simulink model "xEMU_SimulationModel3_rule1"  (R2017b)
settings: Solver=ode4  StartTime=0.0  StopTime=8192  FixedStep=0.01  RelTol=1e-3
undefined symbols (not defined in the file): a1, a2, a3, a4, ACO, BAT, Battery, DCT, DRT, EMS, ENV, Fahrzyklus_VS_modell, height_BAT, leistung, lib_bat, Maximum, Maximum_position, Num_cells, P_FC_max_long, P_FC_min_long, P_FC_step_max, Pbat_charge_max, Pbat_discharge_max, Pfc_max, Pfc_min, SOC_tar, time_peaks, TRM, velocity_peaks
libraries: simulink x5
(part 6 of 15)

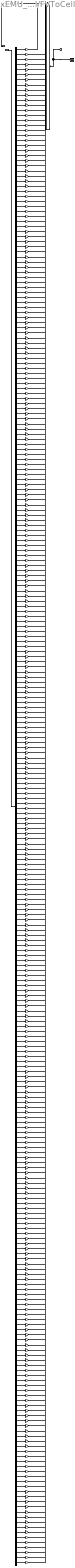
== system xEMU_SimulationModel3_rule1/Battery (BAT)_mittel/Battery/Thermal/FVToCell ==
  T_FV : Inport
  AddCell1 : Sum  Inputs=<binary blob, 300 chars, not shown>
  Demux : Demux  Outputs=300
  Scope : Scope
  T_FV_{1..300} (300 alike) : Gain  Gain=0.0033333  SaturateOnIntegerOverflow=on  OutDataTypeStr=Inherit: Same as input  ParamDataTypeStr=Inherit: Same as input
  Out1 : Outport
  tag scope: T_CellElement1=scoped
  wires:
  T_FV/1 -> Demux/1
  Demux/1 -> T_FV_1/1
  Demux/2 -> T_FV_2/1
  Demux/3 -> T_FV_3/1
  Demux/4 -> T_FV_4/1
  Demux/5 -> T_FV_5/1
  Demux/6 -> T_FV_6/1
  Demux/7 -> T_FV_7/1
  Demux/8 -> T_FV_8/1
  Demux/9 -> T_FV_9/1
  Demux/10 -> T_FV_10/1
  Demux/11 -> T_FV_11/1
  Demux/12 -> T_FV_12/1
  Demux/13 -> T_FV_13/1
  Demux/14 -> T_FV_14/1
  Demux/15 -> T_FV_15/1
  Demux/16 -> T_FV_16/1
  Demux/17 -> T_FV_17/1
  Demux/18 -> T_FV_18/1
  Demux/19 -> T_FV_19/1
  Demux/20 -> T_FV_20/1
  Demux/21 -> T_FV_21/1
  Demux/22 -> T_FV_22/1
  Demux/23 -> T_FV_23/1
  Demux/24 -> T_FV_24/1
  Demux/25 -> T_FV_25/1
  Demux/26 -> T_FV_26/1
  Demux/27 -> T_FV_27/1
  Demux/28 -> T_FV_28/1
  Demux/29 -> T_FV_29/1
  Demux/30 -> T_FV_30/1
  Demux/31 -> T_FV_31/1
  Demux/32 -> T_FV_32/1
  Demux/33 -> T_FV_33/1
  Demux/34 -> T_FV_34/1
  Demux/35 -> T_FV_35/1
  Demux/36 -> T_FV_36/1
  Demux/37 -> T_FV_37/1
  Demux/38 -> T_FV_38/1
  Demux/39 -> T_FV_39/1
  Demux/40 -> T_FV_40/1
  Demux/41 -> T_FV_41/1
  Demux/42 -> T_FV_42/1
  Demux/43 -> T_FV_43/1
  Demux/44 -> T_FV_44/1
  Demux/45 -> T_FV_45/1
  Demux/46 -> T_FV_46/1
  Demux/47 -> T_FV_47/1
  Demux/48 -> T_FV_48/1
  Demux/49 -> T_FV_49/1
  Demux/50 -> T_FV_50/1
  Demux/51 -> T_FV_51/1
  Demux/52 -> T_FV_52/1
  Demux/53 -> T_FV_53/1
  Demux/54 -> T_FV_54/1
  Demux/55 -> T_FV_55/1
  Demux/56 -> T_FV_56/1
  Demux/57 -> T_FV_57/1
  Demux/58 -> T_FV_58/1
  Demux/59 -> T_FV_59/1
  Demux/60 -> T_FV_60/1
  Demux/61 -> T_FV_61/1
  Demux/62 -> T_FV_62/1
  Demux/63 -> T_FV_63/1
  Demux/64 -> T_FV_64/1
  Demux/65 -> T_FV_65/1
  Demux/66 -> T_FV_66/1
  Demux/67 -> T_FV_67/1
  Demux/68 -> T_FV_68/1
  Demux/69 -> T_FV_69/1
  Demux/70 -> T_FV_70/1
  Demux/71 -> T_FV_71/1
  Demux/72 -> T_FV_72/1
  Demux/73 -> T_FV_73/1
  Demux/74 -> T_FV_74/1
  Demux/75 -> T_FV_75/1
  Demux/76 -> T_FV_76/1
  Demux/77 -> T_FV_77/1
  Demux/78 -> T_FV_78/1
  Demux/79 -> T_FV_79/1
  Demux/80 -> T_FV_80/1
  Demux/81 -> T_FV_81/1
  Demux/82 -> T_FV_82/1
  Demux/83 -> T_FV_83/1
  Demux/84 -> T_FV_84/1
  Demux/85 -> T_FV_85/1
  Demux/86 -> T_FV_86/1
  Demux/87 -> T_FV_87/1
  Demux/88 -> T_FV_88/1
  Demux/89 -> T_FV_89/1
  Demux/90 -> T_FV_90/1
  Demux/91 -> T_FV_91/1
  Demux/92 -> T_FV_92/1
  Demux/93 -> T_FV_93/1
  Demux/94 -> T_FV_94/1
  Demux/95 -> T_FV_95/1
  Demux/96 -> T_FV_96/1
  Demux/97 -> T_FV_97/1
  Demux/98 -> T_FV_98/1
  Demux/99 -> T_FV_99/1
  Demux/100 -> T_FV_100/1
  Demux/101 -> T_FV_101/1
  Demux/102 -> T_FV_102/1
  Demux/103 -> T_FV_103/1
  Demux/104 -> T_FV_104/1
  Demux/105 -> T_FV_105/1
  Demux/106 -> T_FV_106/1
  Demux/107 -> T_FV_107/1
  Demux/108 -> T_FV_108/1
  Demux/109 -> T_FV_109/1
  Demux/110 -> T_FV_110/1
  Demux/111 -> T_FV_111/1
  Demux/112 -> T_FV_112/1
  Demux/113 -> T_FV_113/1
  Demux/114 -> T_FV_114/1
  Demux/115 -> T_FV_115/1
  Demux/116 -> T_FV_116/1
  Demux/117 -> T_FV_117/1
  Demux/118 -> T_FV_118/1
  Demux/119 -> T_FV_119/1
  Demux/120 -> T_FV_120/1
  Demux/121 -> T_FV_121/1
  Demux/122 -> T_FV_122/1
  Demux/123 -> T_FV_123/1
  Demux/124 -> T_FV_124/1
  Demux/125 -> T_FV_125/1
  Demux/126 -> T_FV_126/1
  Demux/127 -> T_FV_127/1
  Demux/128 -> T_FV_128/1
  Demux/129 -> T_FV_129/1
  Demux/130 -> T_FV_130/1
  Demux/131 -> T_FV_131/1
  Demux/132 -> T_FV_132/1
  Demux/133 -> T_FV_133/1
  Demux/134 -> T_FV_134/1
  Demux/135 -> T_FV_135/1
  Demux/136 -> T_FV_136/1
  Demux/137 -> T_FV_137/1
  Demux/138 -> T_FV_138/1
  Demux/139 -> T_FV_139/1
  Demux/140 -> T_FV_140/1
  Demux/141 -> T_FV_141/1
  Demux/142 -> T_FV_142/1
  Demux/143 -> T_FV_143/1
  Demux/144 -> T_FV_144/1
  Demux/145 -> T_FV_145/1
  Demux/146 -> T_FV_146/1
  Demux/147 -> T_FV_147/1
  Demux/148 -> T_FV_148/1
  Demux/149 -> T_FV_149/1
  Demux/150 -> T_FV_150/1
  Demux/151 -> T_FV_151/1
  Demux/152 -> T_FV_152/1
  Demux/153 -> T_FV_153/1
  Demux/154 -> T_FV_154/1
  Demux/155 -> T_FV_155/1
  Demux/156 -> T_FV_156/1
  Demux/157 -> T_FV_157/1
  Demux/158 -> T_FV_158/1
  Demux/159 -> T_FV_159/1
  Demux/160 -> T_FV_160/1
  Demux/161 -> T_FV_161/1
  Demux/162 -> T_FV_162/1
  Demux/163 -> T_FV_163/1
  Demux/164 -> T_FV_164/1
  Demux/165 -> T_FV_165/1
  Demux/166 -> T_FV_166/1
  Demux/167 -> T_FV_167/1
  Demux/168 -> T_FV_168/1
  Demux/169 -> T_FV_169/1
  Demux/170 -> T_FV_170/1
  Demux/171 -> T_FV_171/1
  Demux/172 -> T_FV_172/1
  Demux/173 -> T_FV_173/1
  Demux/174 -> T_FV_174/1
  Demux/175 -> T_FV_175/1
  Demux/176 -> T_FV_176/1
  Demux/177 -> T_FV_177/1
  Demux/178 -> T_FV_178/1
  Demux/179 -> T_FV_179/1
  Demux/180 -> T_FV_180/1
  Demux/181 -> T_FV_181/1
  Demux/182 -> T_FV_182/1
  Demux/183 -> T_FV_183/1
  Demux/184 -> T_FV_184/1
  Demux/185 -> T_FV_185/1
  Demux/186 -> T_FV_186/1
  Demux/187 -> T_FV_187/1
  Demux/188 -> T_FV_188/1
  Demux/189 -> T_FV_189/1
  Demux/190 -> T_FV_190/1
  Demux/191 -> T_FV_191/1
  Demux/192 -> T_FV_192/1
  Demux/193 -> T_FV_193/1
  Demux/194 -> T_FV_194/1
  Demux/195 -> T_FV_195/1
  Demux/196 -> T_FV_196/1
  Demux/197 -> T_FV_197/1
  Demux/198 -> T_FV_198/1
  Demux/199 -> T_FV_199/1
  Demux/200 -> T_FV_200/1
  Demux/201 -> T_FV_201/1
  Demux/202 -> T_FV_202/1
  Demux/203 -> T_FV_203/1
  Demux/204 -> T_FV_204/1
  Demux/205 -> T_FV_205/1
  Demux/206 -> T_FV_206/1
  Demux/207 -> T_FV_207/1
  Demux/208 -> T_FV_208/1
  Demux/209 -> T_FV_209/1
  Demux/210 -> T_FV_210/1
  Demux/211 -> T_FV_211/1
  Demux/212 -> T_FV_212/1
  Demux/213 -> T_FV_213/1
  Demux/214 -> T_FV_214/1
  Demux/215 -> T_FV_215/1
  Demux/216 -> T_FV_216/1
  Demux/217 -> T_FV_217/1
  Demux/218 -> T_FV_218/1
  Demux/219 -> T_FV_219/1
  Demux/220 -> T_FV_220/1
  Demux/221 -> T_FV_221/1
  Demux/222 -> T_FV_222/1
  Demux/223 -> T_FV_223/1
  Demux/224 -> T_FV_224/1
  Demux/225 -> T_FV_225/1
  Demux/226 -> T_FV_226/1
  Demux/227 -> T_FV_227/1
  Demux/228 -> T_FV_228/1
  Demux/229 -> T_FV_229/1
  Demux/230 -> T_FV_230/1
  Demux/231 -> T_FV_231/1
  Demux/232 -> T_FV_232/1
  Demux/233 -> T_FV_233/1
  Demux/234 -> T_FV_234/1
  Demux/235 -> T_FV_235/1
  Demux/236 -> T_FV_236/1
  Demux/237 -> T_FV_237/1
  Demux/238 -> T_FV_238/1
  Demux/239 -> T_FV_239/1
  Demux/240 -> T_FV_240/1
  Demux/241 -> T_FV_241/1
  Demux/242 -> T_FV_242/1
  Demux/243 -> T_FV_243/1
  Demux/244 -> T_FV_244/1
  Demux/245 -> T_FV_245/1
  Demux/246 -> T_FV_246/1
  Demux/247 -> T_FV_247/1
  Demux/248 -> T_FV_248/1
  Demux/249 -> T_FV_249/1
  Demux/250 -> T_FV_250/1
  Demux/251 -> T_FV_251/1
  Demux/252 -> T_FV_252/1
  Demux/253 -> T_FV_253/1
  Demux/254 -> T_FV_254/1
  Demux/255 -> T_FV_255/1
  Demux/256 -> T_FV_256/1
  Demux/257 -> T_FV_257/1
  Demux/258 -> T_FV_258/1
  Demux/259 -> T_FV_259/1
  Demux/260 -> T_FV_260/1
  Demux/261 -> T_FV_261/1
  Demux/262 -> T_FV_262/1
  Demux/263 -> T_FV_263/1
  Demux/264 -> T_FV_264/1
  Demux/265 -> T_FV_265/1
  Demux/266 -> T_FV_266/1
  Demux/267 -> T_FV_267/1
  Demux/268 -> T_FV_268/1
  Demux/269 -> T_FV_269/1
  Demux/270 -> T_FV_270/1
  Demux/271 -> T_FV_271/1
  Demux/272 -> T_FV_272/1
  Demux/273 -> T_FV_273/1
  Demux/274 -> T_FV_274/1
  Demux/275 -> T_FV_275/1
  Demux/276 -> T_FV_276/1
  Demux/277 -> T_FV_277/1
  Demux/278 -> T_FV_278/1
  Demux/279 -> T_FV_279/1
  Demux/280 -> T_FV_280/1
  Demux/281 -> T_FV_281/1
  Demux/282 -> T_FV_282/1
  Demux/283 -> T_FV_283/1
  Demux/284 -> T_FV_284/1
  Demux/285 -> T_FV_285/1
  Demux/286 -> T_FV_286/1
  Demux/287 -> T_FV_287/1
  Demux/288 -> T_FV_288/1
  Demux/289 -> T_FV_289/1
  Demux/290 -> T_FV_290/1
  Demux/291 -> T_FV_291/1
  Demux/292 -> T_FV_292/1
  Demux/293 -> T_FV_293/1
  Demux/294 -> T_FV_294/1
  Demux/295 -> T_FV_295/1
  Demux/296 -> T_FV_296/1
  Demux/297 -> T_FV_297/1
  Demux/298 -> T_FV_298/1
  Demux/299 -> T_FV_299/1
  Demux/300 -> T_FV_300/1
  AddCell1/1 -> Scope/1, [T_CellElement1], Out1/1
  T_FV_1/1 -> AddCell1/1
  T_FV_2/1 -> AddCell1/2
  T_FV_3/1 -> AddCell1/3
  T_FV_4/1 -> AddCell1/4
  T_FV_5/1 -> AddCell1/5
  T_FV_6/1 -> AddCell1/6
  T_FV_7/1 -> AddCell1/7
  T_FV_8/1 -> AddCell1/8
  T_FV_9/1 -> AddCell1/9
  T_FV_10/1 -> AddCell1/10
  T_FV_11/1 -> AddCell1/11
  T_FV_12/1 -> AddCell1/12
  T_FV_13/1 -> AddCell1/13
  T_FV_14/1 -> AddCell1/14
  T_FV_15/1 -> AddCell1/15
  T_FV_16/1 -> AddCell1/16
  T_FV_17/1 -> AddCell1/17
  T_FV_18/1 -> AddCell1/18
  T_FV_19/1 -> AddCell1/19
  T_FV_20/1 -> AddCell1/20
  T_FV_21/1 -> AddCell1/21
  T_FV_22/1 -> AddCell1/22
  T_FV_23/1 -> AddCell1/23
  T_FV_24/1 -> AddCell1/24
  T_FV_25/1 -> AddCell1/25
  T_FV_26/1 -> AddCell1/26
  T_FV_27/1 -> AddCell1/27
  T_FV_28/1 -> AddCell1/28
  T_FV_29/1 -> AddCell1/29
  T_FV_30/1 -> AddCell1/30
  T_FV_31/1 -> AddCell1/31
  T_FV_32/1 -> AddCell1/32
  T_FV_33/1 -> AddCell1/33
  T_FV_34/1 -> AddCell1/34
  T_FV_35/1 -> AddCell1/35
  T_FV_36/1 -> AddCell1/36
  T_FV_37/1 -> AddCell1/37
  T_FV_38/1 -> AddCell1/38
  T_FV_39/1 -> AddCell1/39
  T_FV_40/1 -> AddCell1/40
  T_FV_41/1 -> AddCell1/41
  T_FV_42/1 -> AddCell1/42
  T_FV_43/1 -> AddCell1/43
  T_FV_44/1 -> AddCell1/44
  T_FV_45/1 -> AddCell1/45
  T_FV_46/1 -> AddCell1/46
  T_FV_47/1 -> AddCell1/47
  T_FV_48/1 -> AddCell1/48
  T_FV_49/1 -> AddCell1/49
  T_FV_50/1 -> AddCell1/50
  T_FV_51/1 -> AddCell1/51
  T_FV_52/1 -> AddCell1/52
  T_FV_53/1 -> AddCell1/53
  T_FV_54/1 -> AddCell1/54
  T_FV_55/1 -> AddCell1/55
  T_FV_56/1 -> AddCell1/56
  T_FV_57/1 -> AddCell1/57
  T_FV_58/1 -> AddCell1/58
  T_FV_59/1 -> AddCell1/59
  T_FV_60/1 -> AddCell1/60
  T_FV_61/1 -> AddCell1/61
  T_FV_62/1 -> AddCell1/62
  T_FV_63/1 -> AddCell1/63
  T_FV_64/1 -> AddCell1/64
  T_FV_65/1 -> AddCell1/65
  T_FV_66/1 -> AddCell1/66
  T_FV_67/1 -> AddCell1/67
  T_FV_68/1 -> AddCell1/68
  T_FV_69/1 -> AddCell1/69
  T_FV_70/1 -> AddCell1/70
  T_FV_71/1 -> AddCell1/71
  T_FV_72/1 -> AddCell1/72
  T_FV_73/1 -> AddCell1/73
  T_FV_74/1 -> AddCell1/74
  T_FV_75/1 -> AddCell1/75
  T_FV_76/1 -> AddCell1/76
  T_FV_77/1 -> AddCell1/77
  T_FV_78/1 -> AddCell1/78
  T_FV_79/1 -> AddCell1/79
  T_FV_80/1 -> AddCell1/80
  T_FV_81/1 -> AddCell1/81
  T_FV_82/1 -> AddCell1/82
  T_FV_83/1 -> AddCell1/83
  T_FV_84/1 -> AddCell1/84
  T_FV_85/1 -> AddCell1/85
  T_FV_86/1 -> AddCell1/86
  T_FV_87/1 -> AddCell1/87
  T_FV_88/1 -> AddCell1/88
  T_FV_89/1 -> AddCell1/89
  T_FV_90/1 -> AddCell1/90
  T_FV_91/1 -> AddCell1/91
  T_FV_92/1 -> AddCell1/92
  T_FV_93/1 -> AddCell1/93
  T_FV_94/1 -> AddCell1/94
  T_FV_95/1 -> AddCell1/95
  T_FV_96/1 -> AddCell1/96
  T_FV_97/1 -> AddCell1/97
  T_FV_98/1 -> AddCell1/98
  T_FV_99/1 -> AddCell1/99
  T_FV_100/1 -> AddCell1/100
  T_FV_101/1 -> AddCell1/101
  T_FV_102/1 -> AddCell1/102
  T_FV_103/1 -> AddCell1/103
  T_FV_104/1 -> AddCell1/104
  T_FV_105/1 -> AddCell1/105
  T_FV_106/1 -> AddCell1/106
  T_FV_107/1 -> AddCell1/107
  T_FV_108/1 -> AddCell1/108
  T_FV_109/1 -> AddCell1/109
  T_FV_110/1 -> AddCell1/110
  T_FV_111/1 -> AddCell1/111
  T_FV_112/1 -> AddCell1/112
  T_FV_113/1 -> AddCell1/113
  T_FV_114/1 -> AddCell1/114
  T_FV_115/1 -> AddCell1/115
  T_FV_116/1 -> AddCell1/116
  T_FV_117/1 -> AddCell1/117
  T_FV_118/1 -> AddCell1/118
  T_FV_119/1 -> AddCell1/119
  T_FV_120/1 -> AddCell1/120
  T_FV_121/1 -> AddCell1/121
  T_FV_122/1 -> AddCell1/122
  T_FV_123/1 -> AddCell1/123
  T_FV_124/1 -> AddCell1/124
  T_FV_125/1 -> AddCell1/125
  T_FV_126/1 -> AddCell1/126
  T_FV_127/1 -> AddCell1/127
  T_FV_128/1 -> AddCell1/128
  T_FV_129/1 -> AddCell1/129
  T_FV_130/1 -> AddCell1/130
  T_FV_131/1 -> AddCell1/131
  T_FV_132/1 -> AddCell1/132
  T_FV_133/1 -> AddCell1/133
  T_FV_134/1 -> AddCell1/134
  T_FV_135/1 -> AddCell1/135
  T_FV_136/1 -> AddCell1/136
  T_FV_137/1 -> AddCell1/137
  T_FV_138/1 -> AddCell1/138
  T_FV_139/1 -> AddCell1/139
  T_FV_140/1 -> AddCell1/140
  T_FV_141/1 -> AddCell1/141
  T_FV_142/1 -> AddCell1/142
  T_FV_143/1 -> AddCell1/143
  T_FV_144/1 -> AddCell1/144
  T_FV_145/1 -> AddCell1/145
  T_FV_146/1 -> AddCell1/146
  T_FV_147/1 -> AddCell1/147
  T_FV_148/1 -> AddCell1/148
  T_FV_149/1 -> AddCell1/149
  T_FV_150/1 -> AddCell1/150
  T_FV_151/1 -> AddCell1/151
  T_FV_152/1 -> AddCell1/152
  T_FV_153/1 -> AddCell1/153
  T_FV_154/1 -> AddCell1/154
  T_FV_155/1 -> AddCell1/155
  T_FV_156/1 -> AddCell1/156
  T_FV_157/1 -> AddCell1/157
  T_FV_158/1 -> AddCell1/158
  T_FV_159/1 -> AddCell1/159
  T_FV_160/1 -> AddCell1/160
  T_FV_161/1 -> AddCell1/161
  T_FV_162/1 -> AddCell1/162
  T_FV_163/1 -> AddCell1/163
  T_FV_164/1 -> AddCell1/164
  T_FV_165/1 -> AddCell1/165
  T_FV_166/1 -> AddCell1/166
  T_FV_167/1 -> AddCell1/167
  T_FV_168/1 -> AddCell1/168
  T_FV_169/1 -> AddCell1/169
  T_FV_170/1 -> AddCell1/170
  T_FV_171/1 -> AddCell1/171
  T_FV_172/1 -> AddCell1/172
  T_FV_173/1 -> AddCell1/173
  T_FV_174/1 -> AddCell1/174
  T_FV_175/1 -> AddCell1/175
  T_FV_176/1 -> AddCell1/176
  T_FV_177/1 -> AddCell1/177
  T_FV_178/1 -> AddCell1/178
  T_FV_179/1 -> AddCell1/179
  T_FV_180/1 -> AddCell1/180
  T_FV_181/1 -> AddCell1/181
  T_FV_182/1 -> AddCell1/182
  T_FV_183/1 -> AddCell1/183
  T_FV_184/1 -> AddCell1/184
  T_FV_185/1 -> AddCell1/185
  T_FV_186/1 -> AddCell1/186
  T_FV_187/1 -> AddCell1/187
  T_FV_188/1 -> AddCell1/188
  T_FV_189/1 -> AddCell1/189
  T_FV_190/1 -> AddCell1/190
  T_FV_191/1 -> AddCell1/191
  T_FV_192/1 -> AddCell1/192
  T_FV_193/1 -> AddCell1/193
  T_FV_194/1 -> AddCell1/194
  T_FV_195/1 -> AddCell1/195
  T_FV_196/1 -> AddCell1/196
  T_FV_197/1 -> AddCell1/197
  T_FV_198/1 -> AddCell1/198
  T_FV_199/1 -> AddCell1/199
  T_FV_200/1 -> AddCell1/200
  T_FV_201/1 -> AddCell1/201
  T_FV_202/1 -> AddCell1/202
  T_FV_203/1 -> AddCell1/203
  T_FV_204/1 -> AddCell1/204
  T_FV_205/1 -> AddCell1/205
  T_FV_206/1 -> AddCell1/206
  T_FV_207/1 -> AddCell1/207
  T_FV_208/1 -> AddCell1/208
  T_FV_209/1 -> AddCell1/209
  T_FV_210/1 -> AddCell1/210
  T_FV_211/1 -> AddCell1/211
  T_FV_212/1 -> AddCell1/212
  T_FV_213/1 -> AddCell1/213
  T_FV_214/1 -> AddCell1/214
  T_FV_215/1 -> AddCell1/215
  T_FV_216/1 -> AddCell1/216
  T_FV_217/1 -> AddCell1/217
  T_FV_218/1 -> AddCell1/218
  T_FV_219/1 -> AddCell1/219
  T_FV_220/1 -> AddCell1/220
  T_FV_221/1 -> AddCell1/221
  T_FV_222/1 -> AddCell1/222
  T_FV_223/1 -> AddCell1/223
  T_FV_224/1 -> AddCell1/224
  T_FV_225/1 -> AddCell1/225
  T_FV_226/1 -> AddCell1/226
  T_FV_227/1 -> AddCell1/227
  T_FV_228/1 -> AddCell1/228
  T_FV_229/1 -> AddCell1/229
  T_FV_230/1 -> AddCell1/230
  T_FV_231/1 -> AddCell1/231
  T_FV_232/1 -> AddCell1/232
  T_FV_233/1 -> AddCell1/233
  T_FV_234/1 -> AddCell1/234
  T_FV_235/1 -> AddCell1/235
  T_FV_236/1 -> AddCell1/236
  T_FV_237/1 -> AddCell1/237
  T_FV_238/1 -> AddCell1/238
  T_FV_239/1 -> AddCell1/239
  T_FV_240/1 -> AddCell1/240
  T_FV_241/1 -> AddCell1/241
  T_FV_242/1 -> AddCell1/242
  T_FV_243/1 -> AddCell1/243
  T_FV_244/1 -> AddCell1/244
  T_FV_245/1 -> AddCell1/245
  T_FV_246/1 -> AddCell1/246
  T_FV_247/1 -> AddCell1/247
  T_FV_248/1 -> AddCell1/248
  T_FV_249/1 -> AddCell1/249
  T_FV_250/1 -> AddCell1/250
  T_FV_251/1 -> AddCell1/251
  T_FV_252/1 -> AddCell1/252
  T_FV_253/1 -> AddCell1/253
  T_FV_254/1 -> AddCell1/254
  T_FV_255/1 -> AddCell1/255
  T_FV_256/1 -> AddCell1/256
  T_FV_257/1 -> AddCell1/257
  T_FV_258/1 -> AddCell1/258
  T_FV_259/1 -> AddCell1/259
  T_FV_260/1 -> AddCell1/260
  T_FV_261/1 -> AddCell1/261
  T_FV_262/1 -> AddCell1/262
  T_FV_263/1 -> AddCell1/263
  T_FV_264/1 -> AddCell1/264
  T_FV_265/1 -> AddCell1/265
  T_FV_266/1 -> AddCell1/266
  T_FV_267/1 -> AddCell1/267
  T_FV_268/1 -> AddCell1/268
  T_FV_269/1 -> AddCell1/269
  T_FV_270/1 -> AddCell1/270
  T_FV_271/1 -> AddCell1/271
  T_FV_272/1 -> AddCell1/272
  T_FV_273/1 -> AddCell1/273
  T_FV_274/1 -> AddCell1/274
  T_FV_275/1 -> AddCell1/275
  T_FV_276/1 -> AddCell1/276
  T_FV_277/1 -> AddCell1/277
  T_FV_278/1 -> AddCell1/278
  T_FV_279/1 -> AddCell1/279
  T_FV_280/1 -> AddCell1/280
  T_FV_281/1 -> AddCell1/281
  T_FV_282/1 -> AddCell1/282
  T_FV_283/1 -> AddCell1/283
  T_FV_284/1 -> AddCell1/284
  T_FV_285/1 -> AddCell1/285
  T_FV_286/1 -> AddCell1/286
  T_FV_287/1 -> AddCell1/287
  T_FV_288/1 -> AddCell1/288
  T_FV_289/1 -> AddCell1/289
  T_FV_290/1 -> AddCell1/290
  T_FV_291/1 -> AddCell1/291
  T_FV_292/1 -> AddCell1/292
  T_FV_293/1 -> AddCell1/293
  T_FV_294/1 -> AddCell1/294
  T_FV_295/1 -> AddCell1/295
  T_FV_296/1 -> AddCell1/296
  T_FV_297/1 -> AddCell1/297
  T_FV_298/1 -> AddCell1/298
  T_FV_299/1 -> AddCell1/299
  T_FV_300/1 -> AddCell1/300

== system xEMU_SimulationModel3_rule1/Battery (BAT)_mittel/Subsystem1/CellCurrentMatrices/Component0 ==
  ColConst : Constant  Value=0
  RowConst : Constant  Value=0
  Row : Outport
  Col : Outport  Port=2
  Value : Outport  Port=3
  wires:
  ColConst/1 -> Col/1
  RowConst/1 -> Row/1
  [InputCurrent] -> Value/1

== system xEMU_SimulationModel3_rule1/Battery (BAT)_mittel/Subsystem1/CellCurrentMatrices/Component1 ==
  ColConst : Constant  Value=0
  RowConst : Constant  Value=0
  Row : Outport
  Col : Outport  Port=2
  Value : Outport  Port=3
  wires:
  ColConst/1 -> Col/1
  RowConst/1 -> Row/1
  [InputCurrent] -> Value/1

== system xEMU_SimulationModel3_rule1/Battery (BAT)_mittel/Subsystem1/CellVoltageMatrices/Component0 ==
  Add10_1 : Sum
  Add11_1 : Sum
  Add12_1 : Sum
  Add13_1 : Sum
  Add14_1 : Sum
  Add15_1 : Sum
  Add15_4 : Sum
  Add16_1 : Sum
  Add16_3 : Sum
  Add16_4 : Sum
  Add17_1 : Sum
  Add17_3 : Sum
  Add18_1 : Sum
  Add18_3 : Sum
  Add19_1 : Sum
  Add19_2 : Sum
  Add20_1 : Sum
  Add2_1 : Sum
  Add3_1 : Sum
  Add4_1 : Sum
  Add5_1 : Sum
  Add6_1 : Sum
  Add7_1 : Sum
  Add8_1 : Sum
  Add8_4 : Sum
  Add9_1 : Sum
  Add9_8 : Sum
  ColConst : Constant  Value=0
  Const10_10 : Constant
  Const10_4 : Constant  Value=0.5
  Const10_5 : Constant
  Const11_6 : Constant  Value=0.5
  Const11_7 : Constant
  Const15_8 : Constant  Value=0.022993
  Const4_4 : Constant  Value=0.5
  Const5_3 : Constant  Value=2
  Const5_6 : Constant  Value=0.5
  Const6_3 : Constant  Value=2.718
  Const6_5 : Constant  Value=2
  Const7_4 : Constant
  Const7_5 : Constant  Value=2.718
  Const8_3 : Constant  Value=2
  Const8_6 : Constant
  Const9_5 : Constant
  Const9_7 : Constant  Value=2
  Div10_11 : Product  Inputs=*/
  Div11_4 : Product  Inputs=*/
  Div12_6 : Product  Inputs=*/
  Div4_3 : Product  Inputs=*/
  Div5_5 : Product  Inputs=*/
  Div9_6 : Product  Inputs=*/
  Mul10_3 : Product
  Mul11_5 : Product
  Mul12_3 : Product
  Mul13_7 : Product
  Mul14_5 : Product
  Mul14_6 : Product
  Mul15_3 : Product
  Mul15_5 : Product
  Mul15_6 : Product
  Mul16_5 : Product
  Mul17_4 : Product
  Mul6_4 : Product
  Mul7_6 : Product
  Pow11_3 : Math  Operator=pow  SaturateOnIntegerOverflow=on
  Pow12_5 : Math  Operator=pow  SaturateOnIntegerOverflow=on
  Pow5_4 : Math  Operator=pow  SaturateOnIntegerOverflow=on
  Pow6_6 : Math  Operator=pow  SaturateOnIntegerOverflow=on
  Pow7_3 : Math  Operator=pow  SaturateOnIntegerOverflow=on
  Pow8_5 : Math  Operator=pow  SaturateOnIntegerOverflow=on
  RowConst : Constant  Value=0
  Sub10_7 : Sum  Inputs=+-
  Sub11_9 : Sum  Inputs=+-
  Sub13_6 : Sum  Inputs=+-
  Sub14_10 : Sum  Inputs=+-
  Row : Outport
  Col : Outport  Port=2
  Value : Outport  Port=3
  wires:
  ColConst/1 -> Col/1
  RowConst/1 -> Row/1
  Add20_1/1 -> Value/1
  Add19_1/1 -> Add20_1/1
  Add18_1/1 -> Add19_1/1
  Add17_1/1 -> Add18_1/1
  Add16_1/1 -> Add17_1/1
  Add15_1/1 -> Add16_1/1
  Add14_1/1 -> Add15_1/1
  Add13_1/1 -> Add14_1/1
  Add12_1/1 -> Add13_1/1
  Add11_1/1 -> Add12_1/1
  Add10_1/1 -> Add11_1/1
  Add9_1/1 -> Add10_1/1
  Add8_1/1 -> Add9_1/1
  Add7_1/1 -> Add8_1/1
  Add6_1/1 -> Add7_1/1
  Add5_1/1 -> Add6_1/1
  Add4_1/1 -> Add5_1/1
  Add3_1/1 -> Add4_1/1
  Add2_1/1 -> Add3_1/1
  [State1] -> Add2_1/1
  [State2] -> Add2_1/2
  [State3] -> Add3_1/2
  [State4] -> Add4_1/2
  [State5] -> Add5_1/2
  [State6] -> Add6_1/2
  [State7] -> Add7_1/2
  [State8] -> Add8_1/2
  [State9] -> Add9_1/2
  [State10] -> Add10_1/2
  [State11] -> Add11_1/2
  [State12] -> Add12_1/2
  [State13] -> Add13_1/2
  [State14] -> Add14_1/2
  [State15] -> Add15_1/2
  [State16] -> Add16_1/2
  [State17] -> Add17_1/2
  [State18] -> Add18_1/2
  [State19] -> Add19_1/2
  Add19_2/1 -> Add20_1/2
  Add18_3/1 -> Add19_2/1
  Add17_3/1 -> Add18_3/1
  Add16_3/1 -> Add17_3/1
  Mul15_3/1 -> Add16_3/1
  [InputCurrent] -> Mul15_3/1
  [ID1_ObjR] -> Mul15_3/2
  Add15_4/1 -> Add16_3/2
  Mul14_5/1 -> Add15_4/1
  [InputCurrent] -> Mul14_5/1
  [ID0_ObjR] -> Mul14_5/2
  Mul14_6/1 -> Add15_4/2
  [InputCurrent] -> Mul14_6/1
  Sub13_6/1 -> Mul14_6/2
  Mul12_3/1 -> Sub13_6/1
  Pow11_3/1 -> Mul12_3/1
  Mul10_3/1 -> Pow11_3/1
  [ID4_ObjCT] -> Mul10_3/1
  [ID4_ObjMP] -> Mul10_3/2
  Const10_4/1 -> Pow11_3/2
  Div11_4/1 -> Mul12_3/2
  Const10_5/1 -> Div11_4/1
  Sub10_7/1 -> Div11_4/2
  Const9_5/1 -> Sub10_7/1
  Div9_6/1 -> Sub10_7/2
  Const8_3/1 -> Div9_6/1
  Add8_4/1 -> Div9_6/2
  Pow7_3/1 -> Add8_4/1
  Const6_3/1 -> Pow7_3/1
  Mul6_4/1 -> Pow7_3/2
  Const5_3/1 -> Mul6_4/1
  Pow5_4/1 -> Mul6_4/2
  Div4_3/1 -> Pow5_4/1
  [ID4_ObjMP] -> Div4_3/1
  [ID4_ObjCT] -> Div4_3/2
  Const4_4/1 -> Pow5_4/2
  Const7_4/1 -> Add8_4/2
  [ID4_ObjCT] -> Sub13_6/2
  Add16_4/1 -> Add17_3/2
  Mul15_5/1 -> Add16_4/1
  [InputCurrent] -> Mul15_5/1
  [ID0_ObjR] -> Mul15_5/2
  Mul15_6/1 -> Add16_4/2
  [InputCurrent] -> Mul15_6/1
  Sub14_10/1 -> Mul15_6/2
  Mul13_7/1 -> Sub14_10/1
  Pow12_5/1 -> Mul13_7/1
  Mul11_5/1 -> Pow12_5/1
  [ID5_ObjCT] -> Mul11_5/1
  [ID5_ObjMP] -> Mul11_5/2
  Const11_6/1 -> Pow12_5/2
  Div12_6/1 -> Mul13_7/2
  Const11_7/1 -> Div12_6/1
  Sub11_9/1 -> Div12_6/2
  Const10_10/1 -> Sub11_9/1
  Div10_11/1 -> Sub11_9/2
  Const9_7/1 -> Div10_11/1
  Add9_8/1 -> Div10_11/2
  Pow8_5/1 -> Add9_8/1
  Const7_5/1 -> Pow8_5/1
  Mul7_6/1 -> Pow8_5/2
  Const6_5/1 -> Mul7_6/1
  Pow6_6/1 -> Mul7_6/2
  Div5_5/1 -> Pow6_6/1
  [ID5_ObjMP] -> Div5_5/1
  [ID5_ObjCT] -> Div5_5/2
  Const5_6/1 -> Pow6_6/2
  Const8_6/1 -> Add9_8/2
  [ID5_ObjCT] -> Sub14_10/2
  Mul17_4/1 -> Add18_3/2
  Mul16_5/1 -> Mul17_4/1
  [InputCurrent] -> Mul16_5/1
  Const15_8/1 -> Mul16_5/2
  [ID6_ObjR] -> Mul17_4/2
  [ID7_ObjV] -> Add19_2/2

== system xEMU_SimulationModel3_rule1/Battery (BAT)_mittel/Subsystem1/CellVoltageMatrices/Component1 ==
  Add10_1 : Sum
  Add11_1 : Sum
  Add12_1 : Sum
  Add13_1 : Sum
  Add14_1 : Sum
  Add15_1 : Sum
  Add15_4 : Sum
  Add16_1 : Sum
  Add16_3 : Sum
  Add16_4 : Sum
  Add17_1 : Sum
  Add17_3 : Sum
  Add18_1 : Sum
  Add18_3 : Sum
  Add19_1 : Sum
  Add19_2 : Sum
  Add20_1 : Sum
  Add2_1 : Sum
  Add3_1 : Sum
  Add4_1 : Sum
  Add5_1 : Sum
  Add6_1 : Sum
  Add7_1 : Sum
  Add8_1 : Sum
  Add8_4 : Sum
  Add9_1 : Sum
  Add9_8 : Sum
  ColConst : Constant  Value=0
  Const10_10 : Constant
  Const10_4 : Constant  Value=0.5
  Const10_5 : Constant
  Const11_6 : Constant  Value=0.5
  Const11_7 : Constant
  Const15_8 : Constant  Value=0.022993
  Const4_4 : Constant  Value=0.5
  Const5_3 : Constant  Value=2
  Const5_6 : Constant  Value=0.5
  Const6_3 : Constant  Value=2.718
  Const6_5 : Constant  Value=2
  Const7_4 : Constant
  Const7_5 : Constant  Value=2.718
  Const8_3 : Constant  Value=2
  Const8_6 : Constant
  Const9_5 : Constant
  Const9_7 : Constant  Value=2
  Div10_11 : Product  Inputs=*/
  Div11_4 : Product  Inputs=*/
  Div12_6 : Product  Inputs=*/
  Div4_3 : Product  Inputs=*/
  Div5_5 : Product  Inputs=*/
  Div9_6 : Product  Inputs=*/
  Mul10_3 : Product
  Mul11_5 : Product
  Mul12_3 : Product
  Mul13_7 : Product
  Mul14_5 : Product
  Mul14_6 : Product
  Mul15_3 : Product
  Mul15_5 : Product
  Mul15_6 : Product
  Mul16_5 : Product
  Mul17_4 : Product
  Mul6_4 : Product
  Mul7_6 : Product
  Pow11_3 : Math  Operator=pow  SaturateOnIntegerOverflow=on
  Pow12_5 : Math  Operator=pow  SaturateOnIntegerOverflow=on
  Pow5_4 : Math  Operator=pow  SaturateOnIntegerOverflow=on
  Pow6_6 : Math  Operator=pow  SaturateOnIntegerOverflow=on
  Pow7_3 : Math  Operator=pow  SaturateOnIntegerOverflow=on
  Pow8_5 : Math  Operator=pow  SaturateOnIntegerOverflow=on
  RowConst : Constant  Value=0
  Sub10_7 : Sum  Inputs=+-
  Sub11_9 : Sum  Inputs=+-
  Sub13_6 : Sum  Inputs=+-
  Sub14_10 : Sum  Inputs=+-
  Row : Outport
  Col : Outport  Port=2
  Value : Outport  Port=3
  wires:
  ColConst/1 -> Col/1
  RowConst/1 -> Row/1
  Add20_1/1 -> Value/1
  Add19_1/1 -> Add20_1/1
  Add18_1/1 -> Add19_1/1
  Add17_1/1 -> Add18_1/1
  Add16_1/1 -> Add17_1/1
  Add15_1/1 -> Add16_1/1
  Add14_1/1 -> Add15_1/1
  Add13_1/1 -> Add14_1/1
  Add12_1/1 -> Add13_1/1
  Add11_1/1 -> Add12_1/1
  Add10_1/1 -> Add11_1/1
  Add9_1/1 -> Add10_1/1
  Add8_1/1 -> Add9_1/1
  Add7_1/1 -> Add8_1/1
  Add6_1/1 -> Add7_1/1
  Add5_1/1 -> Add6_1/1
  Add4_1/1 -> Add5_1/1
  Add3_1/1 -> Add4_1/1
  Add2_1/1 -> Add3_1/1
  [State1] -> Add2_1/1
  [State2] -> Add2_1/2
  [State3] -> Add3_1/2
  [State4] -> Add4_1/2
  [State5] -> Add5_1/2
  [State6] -> Add6_1/2
  [State7] -> Add7_1/2
  [State8] -> Add8_1/2
  [State9] -> Add9_1/2
  [State10] -> Add10_1/2
  [State11] -> Add11_1/2
  [State12] -> Add12_1/2
  [State13] -> Add13_1/2
  [State14] -> Add14_1/2
  [State15] -> Add15_1/2
  [State16] -> Add16_1/2
  [State17] -> Add17_1/2
  [State18] -> Add18_1/2
  [State19] -> Add19_1/2
  Add19_2/1 -> Add20_1/2
  Add18_3/1 -> Add19_2/1
  Add17_3/1 -> Add18_3/1
  Add16_3/1 -> Add17_3/1
  Mul15_3/1 -> Add16_3/1
  [InputCurrent] -> Mul15_3/1
  [ID1_ObjR] -> Mul15_3/2
  Add15_4/1 -> Add16_3/2
  Mul14_5/1 -> Add15_4/1
  [InputCurrent] -> Mul14_5/1
  [ID0_ObjR] -> Mul14_5/2
  Mul14_6/1 -> Add15_4/2
  [InputCurrent] -> Mul14_6/1
  Sub13_6/1 -> Mul14_6/2
  Mul12_3/1 -> Sub13_6/1
  Pow11_3/1 -> Mul12_3/1
  Mul10_3/1 -> Pow11_3/1
  [ID4_ObjCT] -> Mul10_3/1
  [ID4_ObjMP] -> Mul10_3/2
  Const10_4/1 -> Pow11_3/2
  Div11_4/1 -> Mul12_3/2
  Const10_5/1 -> Div11_4/1
  Sub10_7/1 -> Div11_4/2
  Const9_5/1 -> Sub10_7/1
  Div9_6/1 -> Sub10_7/2
  Const8_3/1 -> Div9_6/1
  Add8_4/1 -> Div9_6/2
  Pow7_3/1 -> Add8_4/1
  Const6_3/1 -> Pow7_3/1
  Mul6_4/1 -> Pow7_3/2
  Const5_3/1 -> Mul6_4/1
  Pow5_4/1 -> Mul6_4/2
  Div4_3/1 -> Pow5_4/1
  [ID4_ObjMP] -> Div4_3/1
  [ID4_ObjCT] -> Div4_3/2
  Const4_4/1 -> Pow5_4/2
  Const7_4/1 -> Add8_4/2
  [ID4_ObjCT] -> Sub13_6/2
  Add16_4/1 -> Add17_3/2
  Mul15_5/1 -> Add16_4/1
  [InputCurrent] -> Mul15_5/1
  [ID0_ObjR] -> Mul15_5/2
  Mul15_6/1 -> Add16_4/2
  [InputCurrent] -> Mul15_6/1
  Sub14_10/1 -> Mul15_6/2
  Mul13_7/1 -> Sub14_10/1
  Pow12_5/1 -> Mul13_7/1
  Mul11_5/1 -> Pow12_5/1
  [ID5_ObjCT] -> Mul11_5/1
  [ID5_ObjMP] -> Mul11_5/2
  Const11_6/1 -> Pow12_5/2
  Div12_6/1 -> Mul13_7/2
  Const11_7/1 -> Div12_6/1
  Sub11_9/1 -> Div12_6/2
  Const10_10/1 -> Sub11_9/1
  Div10_11/1 -> Sub11_9/2
  Const9_7/1 -> Div10_11/1
  Add9_8/1 -> Div10_11/2
  Pow8_5/1 -> Add9_8/1
  Const7_5/1 -> Pow8_5/1
  Mul7_6/1 -> Pow8_5/2
  Const6_5/1 -> Mul7_6/1
  Pow6_6/1 -> Mul7_6/2
  Div5_5/1 -> Pow6_6/1
  [ID5_ObjMP] -> Div5_5/1
  [ID5_ObjCT] -> Div5_5/2
  Const5_6/1 -> Pow6_6/2
  Const8_6/1 -> Add9_8/2
  [ID5_ObjCT] -> Sub14_10/2
  Mul17_4/1 -> Add18_3/2
  Mul16_5/1 -> Mul17_4/1
  [InputCurrent] -> Mul16_5/1
  Const15_8/1 -> Mul16_5/2
  [ID6_ObjR] -> Mul17_4/2
  [ID7_ObjV] -> Add19_2/2

== system xEMU_SimulationModel3_rule1/Battery (BAT)_mittel/Subsystem1/ElectricalCircuit/Cellelement_Elem1 ==
  OhmicResistance_Elem1 : Subsystem
  ParallelRC_Elem5 : Subsystem
  ParallelRC_Elem6 : Subsystem
  Rmphn_Elem2 : Subsystem
  Rmphn_Elem3 : Subsystem
  SoC : Integrator  InitialCondition=80  LimitOutput=on  UpperSaturationLimit=100  LowerSaturationLimit=0
  SoCFactor : Gain  Gain=0.0012171
  SphericalDiffusion_Elem4 : Subsystem
  VoltageSource_Elem7 : Subsystem
  Out1 : Outport
  wires:
  [I_CellElement1] -> SoCFactor/1
  SoCFactor/1 -> SoC/1
  [T_CellElement1] -> ParallelRC_Elem6/1(T), VoltageSource_Elem7/1(T), ParallelRC_Elem5/1(T), SphericalDiffusion_Elem4/1(T), Rmphn_Elem3/1(T), Rmphn_Elem2/1(T), OhmicResistance_Elem1/1(T)
  SoC/1 -> Out1/1, ParallelRC_Elem6/2(SoC), VoltageSource_Elem7/2(SoC), ParallelRC_Elem5/2(SoC), SphericalDiffusion_Elem4/2(SoC), Rmphn_Elem3/2(SoC), Rmphn_Elem2/2(SoC), OhmicResistance_Elem1/2(SoC)

== system xEMU_SimulationModel3_rule1/Battery (BAT)_mittel/Subsystem1/MatrixAxC/StateComponent0 ==
  Add5_1 : Sum
  ColConst : Constant  Value=0
  Const1_1 : Constant  Value=-1.000000
  Const1_5 : Constant  Value=0.991746
  Const1_6 : Constant  Value=0.991451
  Const2_2 : Constant  Value=0.991451
  Div2_1 : Product  Inputs=*/
  Div2_3 : Product  Inputs=*/
  Div2_4 : Product  Inputs=*/
  Div3_2 : Product  Inputs=*/
  Integrator : Integrator
  Mul3_4 : Product
  Mul4_1 : Product
  Mul4_2 : Product
  RowConst : Constant  Value=0
  Row : Outport
  Col : Outport  Port=2
  tag scope: State1=global
  wires:
  Integrator/1 -> [State1]
  ColConst/1 -> Col/1
  RowConst/1 -> Row/1
  Add5_1/1 -> Integrator/1
  Mul4_1/1 -> Add5_1/1
  [State1] -> Mul4_1/1
  Div3_2/1 -> Mul4_1/2
  Div2_1/1 -> Div3_2/1
  Const1_1/1 -> Div2_1/1
  [ID6_ObjTau] -> Div2_1/2
  Const2_2/1 -> Div3_2/2
  Mul4_2/1 -> Add5_1/2
  [InputCurrent] -> Mul4_2/1
  Mul3_4/1 -> Mul4_2/2
  Div2_3/1 -> Mul3_4/1
  [ID6_ObjR] -> Div2_3/1
  [ID6_ObjTau] -> Div2_3/2
  Div2_4/1 -> Mul3_4/2
  Const1_5/1 -> Div2_4/1
  Const1_6/1 -> Div2_4/2

== system xEMU_SimulationModel3_rule1/Battery (BAT)_mittel/Subsystem1/MatrixAxC/StateComponent1 ==
  Add5_1 : Sum
  ColConst : Constant  Value=0
  Const1_1 : Constant  Value=-1.000000
  Const1_5 : Constant  Value=0.335190
  Const1_6 : Constant  Value=0.335870
  Const2_2 : Constant  Value=0.335870
  Div2_1 : Product  Inputs=*/
  Div2_3 : Product  Inputs=*/
  Div2_4 : Product  Inputs=*/
  Div3_2 : Product  Inputs=*/
  Integrator : Integrator
  Mul3_4 : Product
  Mul4_1 : Product
  Mul4_2 : Product
  RowConst : Constant
  Row : Outport
  Col : Outport  Port=2
  tag scope: State2=global
  wires:
  Integrator/1 -> [State2]
  ColConst/1 -> Col/1
  RowConst/1 -> Row/1
  Add5_1/1 -> Integrator/1
  Mul4_1/1 -> Add5_1/1
  [State2] -> Mul4_1/1
  Div3_2/1 -> Mul4_1/2
  Div2_1/1 -> Div3_2/1
  Const1_1/1 -> Div2_1/1
  [ID6_ObjTau] -> Div2_1/2
  Const2_2/1 -> Div3_2/2
  Mul4_2/1 -> Add5_1/2
  [InputCurrent] -> Mul4_2/1
  Mul3_4/1 -> Mul4_2/2
  Div2_3/1 -> Mul3_4/1
  [ID6_ObjR] -> Div2_3/1
  [ID6_ObjTau] -> Div2_3/2
  Div2_4/1 -> Mul3_4/2
  Const1_5/1 -> Div2_4/1
  Const1_6/1 -> Div2_4/2

== system xEMU_SimulationModel3_rule1/Battery (BAT)_mittel/Subsystem1/MatrixAxC/StateComponent10 ==
  Add5_1 : Sum
  ColConst : Constant  Value=0
  Const1_1 : Constant  Value=-1.000000
  Const1_5 : Constant  Value=0.020606
  Const1_6 : Constant  Value=0.004354
  Const2_2 : Constant  Value=0.004354
  Div2_1 : Product  Inputs=*/
  Div2_3 : Product  Inputs=*/
  Div2_4 : Product  Inputs=*/
  Div3_2 : Product  Inputs=*/
  Integrator : Integrator
  Mul3_4 : Product
  Mul4_1 : Product
  Mul4_2 : Product
  RowConst : Constant  Value=10
  Row : Outport
  Col : Outport  Port=2
  tag scope: State11=global
  wires:
  Integrator/1 -> [State11]
  ColConst/1 -> Col/1
  RowConst/1 -> Row/1
  Add5_1/1 -> Integrator/1
  Mul4_1/1 -> Add5_1/1
  [State11] -> Mul4_1/1
  Div3_2/1 -> Mul4_1/2
  Div2_1/1 -> Div3_2/1
  Const1_1/1 -> Div2_1/1
  [ID6_ObjTau] -> Div2_1/2
  Const2_2/1 -> Div3_2/2
  Mul4_2/1 -> Add5_1/2
  [InputCurrent] -> Mul4_2/1
  Mul3_4/1 -> Mul4_2/2
  Div2_3/1 -> Mul3_4/1
  [ID6_ObjR] -> Div2_3/1
  [ID6_ObjTau] -> Div2_3/2
  Div2_4/1 -> Mul3_4/2
  Const1_5/1 -> Div2_4/1
  Const1_6/1 -> Div2_4/2

== system xEMU_SimulationModel3_rule1/Battery (BAT)_mittel/Subsystem1/MatrixAxC/StateComponent11 ==
  Add5_1 : Sum
  ColConst : Constant  Value=0
  Const1_1 : Constant  Value=-1.000000
  Const1_5 : Constant  Value=0.016393
  Const1_6 : Constant  Value=0.002781
  Const2_2 : Constant  Value=0.002781
  Div2_1 : Product  Inputs=*/
  Div2_3 : Product  Inputs=*/
  Div2_4 : Product  Inputs=*/
  Div3_2 : Product  Inputs=*/
  Integrator : Integrator
  Mul3_4 : Product
  Mul4_1 : Product
  Mul4_2 : Product
  RowConst : Constant  Value=11
  Row : Outport
  Col : Outport  Port=2
  tag scope: State12=global
  wires:
  Integrator/1 -> [State12]
  ColConst/1 -> Col/1
  RowConst/1 -> Row/1
  Add5_1/1 -> Integrator/1
  Mul4_1/1 -> Add5_1/1
  [State12] -> Mul4_1/1
  Div3_2/1 -> Mul4_1/2
  Div2_1/1 -> Div3_2/1
  Const1_1/1 -> Div2_1/1
  [ID6_ObjTau] -> Div2_1/2
  Const2_2/1 -> Div3_2/2
  Mul4_2/1 -> Add5_1/2
  [InputCurrent] -> Mul4_2/1
  Mul3_4/1 -> Mul4_2/2
  Div2_3/1 -> Mul3_4/1
  [ID6_ObjR] -> Div2_3/1
  [ID6_ObjTau] -> Div2_3/2
  Div2_4/1 -> Mul3_4/2
  Const1_5/1 -> Div2_4/1
  Const1_6/1 -> Div2_4/2

== system xEMU_SimulationModel3_rule1/Battery (BAT)_mittel/Subsystem1/MatrixAxC/StateComponent12 ==
  Add5_1 : Sum
  ColConst : Constant  Value=0
  Const1_1 : Constant  Value=-1.000000
  Const1_5 : Constant  Value=0.013339
  Const1_6 : Constant  Value=0.001779
  Const2_2 : Constant  Value=0.001779
  Div2_1 : Product  Inputs=*/
  Div2_3 : Product  Inputs=*/
  Div2_4 : Product  Inputs=*/
  Div3_2 : Product  Inputs=*/
  Integrator : Integrator
  Mul3_4 : Product
  Mul4_1 : Product
  Mul4_2 : Product
  RowConst : Constant  Value=12
  Row : Outport
  Col : Outport  Port=2
  tag scope: State13=global
  wires:
  Integrator/1 -> [State13]
  ColConst/1 -> Col/1
  RowConst/1 -> Row/1
  Add5_1/1 -> Integrator/1
  Mul4_1/1 -> Add5_1/1
  [State13] -> Mul4_1/1
  Div3_2/1 -> Mul4_1/2
  Div2_1/1 -> Div3_2/1
  Const1_1/1 -> Div2_1/1
  [ID6_ObjTau] -> Div2_1/2
  Const2_2/1 -> Div3_2/2
  Mul4_2/1 -> Add5_1/2
  [InputCurrent] -> Mul4_2/1
  Mul3_4/1 -> Mul4_2/2
  Div2_3/1 -> Mul3_4/1
  [ID6_ObjR] -> Div2_3/1
  [ID6_ObjTau] -> Div2_3/2
  Div2_4/1 -> Mul3_4/2
  Const1_5/1 -> Div2_4/1
  Const1_6/1 -> Div2_4/2

== system xEMU_SimulationModel3_rule1/Battery (BAT)_mittel/Subsystem1/MatrixAxC/StateComponent13 ==
  Add5_1 : Sum
  ColConst : Constant  Value=0
  Const1_1 : Constant  Value=-1.000000
  Const1_5 : Constant  Value=0.009631
  Const1_6 : Constant  Value=0.001139
  Const2_2 : Constant  Value=0.001139
  Div2_1 : Product  Inputs=*/
  Div2_3 : Product  Inputs=*/
  Div2_4 : Product  Inputs=*/
  Div3_2 : Product  Inputs=*/
  Integrator : Integrator
  Mul3_4 : Product
  Mul4_1 : Product
  Mul4_2 : Product
  RowConst : Constant  Value=13
  Row : Outport
  Col : Outport  Port=2
  tag scope: State14=global
  wires:
  Integrator/1 -> [State14]
  ColConst/1 -> Col/1
  RowConst/1 -> Row/1
  Add5_1/1 -> Integrator/1
  Mul4_1/1 -> Add5_1/1
  [State14] -> Mul4_1/1
  Div3_2/1 -> Mul4_1/2
  Div2_1/1 -> Div3_2/1
  Const1_1/1 -> Div2_1/1
  [ID6_ObjTau] -> Div2_1/2
  Const2_2/1 -> Div3_2/2
  Mul4_2/1 -> Add5_1/2
  [InputCurrent] -> Mul4_2/1
  Mul3_4/1 -> Mul4_2/2
  Div2_3/1 -> Mul3_4/1
  [ID6_ObjR] -> Div2_3/1
  [ID6_ObjTau] -> Div2_3/2
  Div2_4/1 -> Mul3_4/2
  Const1_5/1 -> Div2_4/1
  Const1_6/1 -> Div2_4/2

== system xEMU_SimulationModel3_rule1/Battery (BAT)_mittel/Subsystem1/MatrixAxC/StateComponent14 ==
  Add5_1 : Sum
  ColConst : Constant  Value=0
  Const1_1 : Constant  Value=-1.000000
  Const1_5 : Constant  Value=0.010562
  Const1_6 : Constant  Value=0.000732
  Const2_2 : Constant  Value=0.000732
  Div2_1 : Product  Inputs=*/
  Div2_3 : Product  Inputs=*/
  Div2_4 : Product  Inputs=*/
  Div3_2 : Product  Inputs=*/
  Integrator : Integrator
  Mul3_4 : Product
  Mul4_1 : Product
  Mul4_2 : Product
  RowConst : Constant  Value=14
  Row : Outport
  Col : Outport  Port=2
  tag scope: State15=global
  wires:
  Integrator/1 -> [State15]
  ColConst/1 -> Col/1
  RowConst/1 -> Row/1
  Add5_1/1 -> Integrator/1
  Mul4_1/1 -> Add5_1/1
  [State15] -> Mul4_1/1
  Div3_2/1 -> Mul4_1/2
  Div2_1/1 -> Div3_2/1
  Const1_1/1 -> Div2_1/1
  [ID6_ObjTau] -> Div2_1/2
  Const2_2/1 -> Div3_2/2
  Mul4_2/1 -> Add5_1/2
  [InputCurrent] -> Mul4_2/1
  Mul3_4/1 -> Mul4_2/2
  Div2_3/1 -> Mul3_4/1
  [ID6_ObjR] -> Div2_3/1
  [ID6_ObjTau] -> Div2_3/2
  Div2_4/1 -> Mul3_4/2
  Const1_5/1 -> Div2_4/1
  Const1_6/1 -> Div2_4/2

== system xEMU_SimulationModel3_rule1/Battery (BAT)_mittel/Subsystem1/MatrixAxC/StateComponent15 ==
  Add5_1 : Sum
  ColConst : Constant  Value=0
  Const1_1 : Constant  Value=-1.000000
  Const1_5 : Constant  Value=0.006255
  Const1_6 : Constant  Value=0.000468
  Const2_2 : Constant  Value=0.000468
  Div2_1 : Product  Inputs=*/
  Div2_3 : Product  Inputs=*/
  Div2_4 : Product  Inputs=*/
  Div3_2 : Product  Inputs=*/
  Integrator : Integrator
  Mul3_4 : Product
  Mul4_1 : Product
  Mul4_2 : Product
  RowConst : Constant  Value=15
  Row : Outport
  Col : Outport  Port=2
  tag scope: State16=global
  wires:
  Integrator/1 -> [State16]
  ColConst/1 -> Col/1
  RowConst/1 -> Row/1
  Add5_1/1 -> Integrator/1
  Mul4_1/1 -> Add5_1/1
  [State16] -> Mul4_1/1
  Div3_2/1 -> Mul4_1/2
  Div2_1/1 -> Div3_2/1
  Const1_1/1 -> Div2_1/1
  [ID6_ObjTau] -> Div2_1/2
  Const2_2/1 -> Div3_2/2
  Mul4_2/1 -> Add5_1/2
  [InputCurrent] -> Mul4_2/1
  Mul3_4/1 -> Mul4_2/2
  Div2_3/1 -> Mul3_4/1
  [ID6_ObjR] -> Div2_3/1
  [ID6_ObjTau] -> Div2_3/2
  Div2_4/1 -> Mul3_4/2
  Const1_5/1 -> Div2_4/1
  Const1_6/1 -> Div2_4/2

== system xEMU_SimulationModel3_rule1/Battery (BAT)_mittel/Subsystem1/MatrixAxC/StateComponent16 ==
  Add5_1 : Sum
  ColConst : Constant  Value=0
  Const1_1 : Constant  Value=-1.000000
  Const1_5 : Constant  Value=0.004664
  Const1_6 : Constant  Value=0.000300
  Const2_2 : Constant  Value=0.000300
  Div2_1 : Product  Inputs=*/
  Div2_3 : Product  Inputs=*/
  Div2_4 : Product  Inputs=*/
  Div3_2 : Product  Inputs=*/
  Integrator : Integrator
  Mul3_4 : Product
  Mul4_1 : Product
  Mul4_2 : Product
  RowConst : Constant  Value=16
  Row : Outport
  Col : Outport  Port=2
  tag scope: State17=global
  wires:
  Integrator/1 -> [State17]
  ColConst/1 -> Col/1
  RowConst/1 -> Row/1
  Add5_1/1 -> Integrator/1
  Mul4_1/1 -> Add5_1/1
  [State17] -> Mul4_1/1
  Div3_2/1 -> Mul4_1/2
  Div2_1/1 -> Div3_2/1
  Const1_1/1 -> Div2_1/1
  [ID6_ObjTau] -> Div2_1/2
  Const2_2/1 -> Div3_2/2
  Mul4_2/1 -> Add5_1/2
  [InputCurrent] -> Mul4_2/1
  Mul3_4/1 -> Mul4_2/2
  Div2_3/1 -> Mul3_4/1
  [ID6_ObjR] -> Div2_3/1
  [ID6_ObjTau] -> Div2_3/2
  Div2_4/1 -> Mul3_4/2
  Const1_5/1 -> Div2_4/1
  Const1_6/1 -> Div2_4/2

== system xEMU_SimulationModel3_rule1/Battery (BAT)_mittel/Subsystem1/MatrixAxC/StateComponent17 ==
  Add5_1 : Sum
  ColConst : Constant  Value=0
  Const1_1 : Constant  Value=1.000000
  Div2_1 : Product  Inputs=*/
  Div4_2 : Product  Inputs=*/
  Integrator : Integrator
  Mul3_3 : Product
  Mul4_1 : Product
  Neg3_2 : Gain  Gain=-1
  RowConst : Constant  Value=17
  Row : Outport
  Col : Outport  Port=2
  tag scope: State18=global
  wires:
  Integrator/1 -> [State18]
  ColConst/1 -> Col/1
  RowConst/1 -> Row/1
  Add5_1/1 -> Integrator/1
  Mul4_1/1 -> Add5_1/1
  [State18] -> Mul4_1/1
  Neg3_2/1 -> Mul4_1/2
  Div2_1/1 -> Neg3_2/1
  Const1_1/1 -> Div2_1/1
  [ID2_ObjTau] -> Div2_1/2
  Div4_2/1 -> Add5_1/2
  Mul3_3/1 -> Div4_2/1
  [InputCurrent] -> Mul3_3/1
  [ID2_ObjR] -> Mul3_3/2
  [ID2_ObjTau] -> Div4_2/2

== system xEMU_SimulationModel3_rule1/Battery (BAT)_mittel/Subsystem1/MatrixAxC/StateComponent18 ==
  Add5_1 : Sum
  ColConst : Constant  Value=0
  Const1_1 : Constant  Value=1.000000
  Div2_1 : Product  Inputs=*/
  Div4_2 : Product  Inputs=*/
  Integrator : Integrator
  Mul3_3 : Product
  Mul4_1 : Product
  Neg3_2 : Gain  Gain=-1
  RowConst : Constant  Value=18
  Row : Outport
  Col : Outport  Port=2
  tag scope: State19=global
  wires:
  Integrator/1 -> [State19]
  ColConst/1 -> Col/1
  RowConst/1 -> Row/1
  Add5_1/1 -> Integrator/1
  Mul4_1/1 -> Add5_1/1
  [State19] -> Mul4_1/1
  Neg3_2/1 -> Mul4_1/2
  Div2_1/1 -> Neg3_2/1
  Const1_1/1 -> Div2_1/1
  [ID3_ObjTau] -> Div2_1/2
  Div4_2/1 -> Add5_1/2
  Mul3_3/1 -> Div4_2/1
  [InputCurrent] -> Mul3_3/1
  [ID3_ObjR] -> Mul3_3/2
  [ID3_ObjTau] -> Div4_2/2

== system xEMU_SimulationModel3_rule1/Battery (BAT)_mittel/Subsystem1/MatrixAxC/StateComponent2 ==
  Add5_1 : Sum
  ColConst : Constant  Value=0
  Const1_1 : Constant  Value=-1.000000
  Const1_5 : Constant  Value=0.172210
  Const1_6 : Constant  Value=0.167580
  Const2_2 : Constant  Value=0.167580
  Div2_1 : Product  Inputs=*/
  Div2_3 : Product  Inputs=*/
  Div2_4 : Product  Inputs=*/
  Div3_2 : Product  Inputs=*/
  Integrator : Integrator
  Mul3_4 : Product
  Mul4_1 : Product
  Mul4_2 : Product
  RowConst : Constant  Value=2
  Row : Outport
  Col : Outport  Port=2
  tag scope: State3=global
  wires:
  Integrator/1 -> [State3]
  ColConst/1 -> Col/1
  RowConst/1 -> Row/1
  Add5_1/1 -> Integrator/1
  Mul4_1/1 -> Add5_1/1
  [State3] -> Mul4_1/1
  Div3_2/1 -> Mul4_1/2
  Div2_1/1 -> Div3_2/1
  Const1_1/1 -> Div2_1/1
  [ID6_ObjTau] -> Div2_1/2
  Const2_2/1 -> Div3_2/2
  Mul4_2/1 -> Add5_1/2
  [InputCurrent] -> Mul4_2/1
  Mul3_4/1 -> Mul4_2/2
  Div2_3/1 -> Mul3_4/1
  [ID6_ObjR] -> Div2_3/1
  [ID6_ObjTau] -> Div2_3/2
  Div2_4/1 -> Mul3_4/2
  Const1_5/1 -> Div2_4/1
  Const1_6/1 -> Div2_4/2

== system xEMU_SimulationModel3_rule1/Battery (BAT)_mittel/Subsystem1/MatrixAxC/StateComponent3 ==
  Add5_1 : Sum
  ColConst : Constant  Value=0
  Const1_1 : Constant  Value=-1.000000
  Const1_5 : Constant  Value=0.099009
  Const1_6 : Constant  Value=0.097920
  Const2_2 : Constant  Value=0.097920
  Div2_1 : Product  Inputs=*/
  Div2_3 : Product  Inputs=*/
  Div2_4 : Product  Inputs=*/
  Div3_2 : Product  Inputs=*/
  Integrator : Integrator
  Mul3_4 : Product
  Mul4_1 : Product
  Mul4_2 : Product
  RowConst : Constant  Value=3
  Row : Outport
  Col : Outport  Port=2
  tag scope: State4=global
  wires:
  Integrator/1 -> [State4]
  ColConst/1 -> Col/1
  RowConst/1 -> Row/1
  Add5_1/1 -> Integrator/1
  Mul4_1/1 -> Add5_1/1
  [State4] -> Mul4_1/1
  Div3_2/1 -> Mul4_1/2
  Div2_1/1 -> Div3_2/1
  Const1_1/1 -> Div2_1/1
  [ID6_ObjTau] -> Div2_1/2
  Const2_2/1 -> Div3_2/2
  Mul4_2/1 -> Add5_1/2
  [InputCurrent] -> Mul4_2/1
  Mul3_4/1 -> Mul4_2/2
  Div2_3/1 -> Mul3_4/1
  [ID6_ObjR] -> Div2_3/1
  [ID6_ObjTau] -> Div2_3/2
  Div2_4/1 -> Mul3_4/2
  Const1_5/1 -> Div2_4/1
  Const1_6/1 -> Div2_4/2

== system xEMU_SimulationModel3_rule1/Battery (BAT)_mittel/Subsystem1/MatrixAxC/StateComponent4 ==
  Add5_1 : Sum
  ColConst : Constant  Value=0
  Const1_1 : Constant  Value=-1.000000
  Const1_5 : Constant  Value=0.089432
  Const1_6 : Constant  Value=0.061684
  Const2_2 : Constant  Value=0.061684
  Div2_1 : Product  Inputs=*/
  Div2_3 : Product  Inputs=*/
  Div2_4 : Product  Inputs=*/
  Div3_2 : Product  Inputs=*/
  Integrator : Integrator
  Mul3_4 : Product
  Mul4_1 : Product
  Mul4_2 : Product
  RowConst : Constant  Value=4
  Row : Outport
  Col : Outport  Port=2
  tag scope: State5=global
  wires:
  Integrator/1 -> [State5]
  ColConst/1 -> Col/1
  RowConst/1 -> Row/1
  Add5_1/1 -> Integrator/1
  Mul4_1/1 -> Add5_1/1
  [State5] -> Mul4_1/1
  Div3_2/1 -> Mul4_1/2
  Div2_1/1 -> Div3_2/1
  Const1_1/1 -> Div2_1/1
  [ID6_ObjTau] -> Div2_1/2
  Const2_2/1 -> Div3_2/2
  Mul4_2/1 -> Add5_1/2
  [InputCurrent] -> Mul4_2/1
  Mul3_4/1 -> Mul4_2/2
  Div2_3/1 -> Mul3_4/1
  [ID6_ObjR] -> Div2_3/1
  [ID6_ObjTau] -> Div2_3/2
  Div2_4/1 -> Mul3_4/2
  Const1_5/1 -> Div2_4/1
  Const1_6/1 -> Div2_4/2

== system xEMU_SimulationModel3_rule1/Battery (BAT)_mittel/Subsystem1/MatrixAxC/StateComponent5 ==
  Add5_1 : Sum
  ColConst : Constant  Value=0
  Const1_1 : Constant  Value=-1.000000
  Const1_5 : Constant  Value=0.062853
  Const1_6 : Constant  Value=0.039662
  Const2_2 : Constant  Value=0.039662
  Div2_1 : Product  Inputs=*/
  Div2_3 : Product  Inputs=*/
  Div2_4 : Product  Inputs=*/
  Div3_2 : Product  Inputs=*/
  Integrator : Integrator
  Mul3_4 : Product
  Mul4_1 : Product
  Mul4_2 : Product
  RowConst : Constant  Value=5
  Row : Outport
  Col : Outport  Port=2
  tag scope: State6=global
  wires:
  Integrator/1 -> [State6]
  ColConst/1 -> Col/1
  RowConst/1 -> Row/1
  Add5_1/1 -> Integrator/1
  Mul4_1/1 -> Add5_1/1
  [State6] -> Mul4_1/1
  Div3_2/1 -> Mul4_1/2
  Div2_1/1 -> Div3_2/1
  Const1_1/1 -> Div2_1/1
  [ID6_ObjTau] -> Div2_1/2
  Const2_2/1 -> Div3_2/2
  Mul4_2/1 -> Add5_1/2
  [InputCurrent] -> Mul4_2/1
  Mul3_4/1 -> Mul4_2/2
  Div2_3/1 -> Mul3_4/1
  [ID6_ObjR] -> Div2_3/1
  [ID6_ObjTau] -> Div2_3/2
  Div2_4/1 -> Mul3_4/2
  Const1_5/1 -> Div2_4/1
  Const1_6/1 -> Div2_4/2

== system xEMU_SimulationModel3_rule1/Battery (BAT)_mittel/Subsystem1/MatrixAxC/StateComponent6 ==
  Add5_1 : Sum
  ColConst : Constant  Value=0
  Const1_1 : Constant  Value=-1.000000
  Const1_5 : Constant  Value=0.043365
  Const1_6 : Constant  Value=0.025741
  Const2_2 : Constant  Value=0.025741
  Div2_1 : Product  Inputs=*/
  Div2_3 : Product  Inputs=*/
  Div2_4 : Product  Inputs=*/
  Div3_2 : Product  Inputs=*/
  Integrator : Integrator
  Mul3_4 : Product
  Mul4_1 : Product
  Mul4_2 : Product
  RowConst : Constant  Value=6
  Row : Outport
  Col : Outport  Port=2
  tag scope: State7=global
  wires:
  Integrator/1 -> [State7]
  ColConst/1 -> Col/1
  RowConst/1 -> Row/1
  Add5_1/1 -> Integrator/1
  Mul4_1/1 -> Add5_1/1
  [State7] -> Mul4_1/1
  Div3_2/1 -> Mul4_1/2
  Div2_1/1 -> Div3_2/1
  Const1_1/1 -> Div2_1/1
  [ID6_ObjTau] -> Div2_1/2
  Const2_2/1 -> Div3_2/2
  Mul4_2/1 -> Add5_1/2
  [InputCurrent] -> Mul4_2/1
  Mul3_4/1 -> Mul4_2/2
  Div2_3/1 -> Mul3_4/1
  [ID6_ObjR] -> Div2_3/1
  [ID6_ObjTau] -> Div2_3/2
  Div2_4/1 -> Mul3_4/2
  Const1_5/1 -> Div2_4/1
  Const1_6/1 -> Div2_4/2

== system xEMU_SimulationModel3_rule1/Battery (BAT)_mittel/Subsystem1/MatrixAxC/StateComponent7 ==
  Add5_1 : Sum
  ColConst : Constant  Value=0
  Const1_1 : Constant  Value=-1.000000
  Const1_5 : Constant  Value=0.040947
  Const1_6 : Constant  Value=0.016677
  Const2_2 : Constant  Value=0.016677
  Div2_1 : Product  Inputs=*/
  Div2_3 : Product  Inputs=*/
  Div2_4 : Product  Inputs=*/
  Div3_2 : Product  Inputs=*/
  Integrator : Integrator
  Mul3_4 : Product
  Mul4_1 : Product
  Mul4_2 : Product
  RowConst : Constant  Value=7
  Row : Outport
  Col : Outport  Port=2
  tag scope: State8=global
  wires:
  Integrator/1 -> [State8]
  ColConst/1 -> Col/1
  RowConst/1 -> Row/1
  Add5_1/1 -> Integrator/1
  Mul4_1/1 -> Add5_1/1
  [State8] -> Mul4_1/1
  Div3_2/1 -> Mul4_1/2
  Div2_1/1 -> Div3_2/1
  Const1_1/1 -> Div2_1/1
  [ID6_ObjTau] -> Div2_1/2
  Const2_2/1 -> Div3_2/2
  Mul4_2/1 -> Add5_1/2
  [InputCurrent] -> Mul4_2/1
  Mul3_4/1 -> Mul4_2/2
  Div2_3/1 -> Mul3_4/1
  [ID6_ObjR] -> Div2_3/1
  [ID6_ObjTau] -> Div2_3/2
  Div2_4/1 -> Mul3_4/2
  Const1_5/1 -> Div2_4/1
  Const1_6/1 -> Div2_4/2

== system xEMU_SimulationModel3_rule1/Battery (BAT)_mittel/Subsystem1/MatrixAxC/StateComponent8 ==
  Add5_1 : Sum
  ColConst : Constant  Value=0
  Const1_1 : Constant  Value=-1.000000
  Const1_5 : Constant  Value=0.035960
  Const1_6 : Constant  Value=0.010685
  Const2_2 : Constant  Value=0.010685
  Div2_1 : Product  Inputs=*/
  Div2_3 : Product  Inputs=*/
  Div2_4 : Product  Inputs=*/
  Div3_2 : Product  Inputs=*/
  Integrator : Integrator
  Mul3_4 : Product
  Mul4_1 : Product
  Mul4_2 : Product
  RowConst : Constant  Value=8
  Row : Outport
  Col : Outport  Port=2
  tag scope: State9=global
  wires:
  Integrator/1 -> [State9]
  ColConst/1 -> Col/1
  RowConst/1 -> Row/1
  Add5_1/1 -> Integrator/1
  Mul4_1/1 -> Add5_1/1
  [State9] -> Mul4_1/1
  Div3_2/1 -> Mul4_1/2
  Div2_1/1 -> Div3_2/1
  Const1_1/1 -> Div2_1/1
  [ID6_ObjTau] -> Div2_1/2
  Const2_2/1 -> Div3_2/2
  Mul4_2/1 -> Add5_1/2
  [InputCurrent] -> Mul4_2/1
  Mul3_4/1 -> Mul4_2/2
  Div2_3/1 -> Mul3_4/1
  [ID6_ObjR] -> Div2_3/1
  [ID6_ObjTau] -> Div2_3/2
  Div2_4/1 -> Mul3_4/2
  Const1_5/1 -> Div2_4/1
  Const1_6/1 -> Div2_4/2

== system xEMU_SimulationModel3_rule1/Battery (BAT)_mittel/Subsystem1/MatrixAxC/StateComponent9 ==
  Add5_1 : Sum
  ColConst : Constant  Value=0
  Const1_1 : Constant  Value=-1.000000
  Const1_5 : Constant  Value=0.025709
  Const1_6 : Constant  Value=0.006818
  Const2_2 : Constant  Value=0.006818
  Div2_1 : Product  Inputs=*/
  Div2_3 : Product  Inputs=*/
  Div2_4 : Product  Inputs=*/
  Div3_2 : Product  Inputs=*/
  Integrator : Integrator
  Mul3_4 : Product
  Mul4_1 : Product
  Mul4_2 : Product
  RowConst : Constant  Value=9
  Row : Outport
  Col : Outport  Port=2
  tag scope: State10=global
  wires:
  Integrator/1 -> [State10]
  ColConst/1 -> Col/1
  RowConst/1 -> Row/1
  Add5_1/1 -> Integrator/1
  Mul4_1/1 -> Add5_1/1
  [State10] -> Mul4_1/1
  Div3_2/1 -> Mul4_1/2
  Div2_1/1 -> Div3_2/1
  Const1_1/1 -> Div2_1/1
  [ID6_ObjTau] -> Div2_1/2
  Const2_2/1 -> Div3_2/2
  Mul4_2/1 -> Add5_1/2
  [InputCurrent] -> Mul4_2/1
  Mul3_4/1 -> Mul4_2/2
  Div2_3/1 -> Mul3_4/1
  [ID6_ObjR] -> Div2_3/1
  [ID6_ObjTau] -> Div2_3/2
  Div2_4/1 -> Mul3_4/2
  Const1_5/1 -> Div2_4/1
  Const1_6/1 -> Div2_4/2
